simulink model "project3"  (R2022b)
settings: Solver=ode4  StartTime=0.0  StopTime=60  FixedStep=0.01  RelTol=1e-3
values from neighbouring files (symbols this model uses):
  Cd = 0.4    [project3_data.m]
  D_ref = 45    [project3_data.m]
  F_grade_const = M * g * sin(theta_rad)    [project3_data.m]
  F_roll_const = Cr * M * g * cos(theta_rad)    [project3_data.m]
  gamma_x = 0.001    [project3_data.m]
  K00 = (F_roll_const + F_grade_const) / K_torque    [project3_data.m]
  K_gap = 0.25    [project3_data.m]
  K_torque = eta_tf * N_tf2 / r_tire    (= 7.93333333333)    [project3_data.m]
  Kr0 = M_eq / (K_torque * tau_m)    (= 189.075630252)    [project3_data.m]
  Kx0 = -M_eq / (K_torque * tau_m)    (= -189.075630252)    [project3_data.m]
  M_eq = M + Mr2    (= 1200)    [project3_data.m]
  tau_m = 0.8    [project3_data.m]
  Te_max = 600    [project3_data.m]
  Te_min = -500    [project3_data.m]
  v_cmd_max = 90/3.6    (= 25)    [project3_data.m]
  v_cmd_min = 0    [project3_data.m]
  vE0 = 50/3.6    (= 13.8888888889)    [project3_data.m]
  xE0 = 0    [project3_data.m]
  xL0 = d0    (= 60)    [project3_data.m]
settings Model: Creator=Forough  LastModifiedBy=Forough

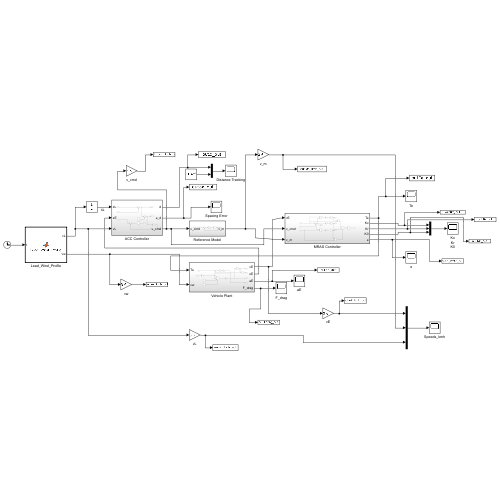
[thumbnail: Simulink's stored preview of the top-level diagram]
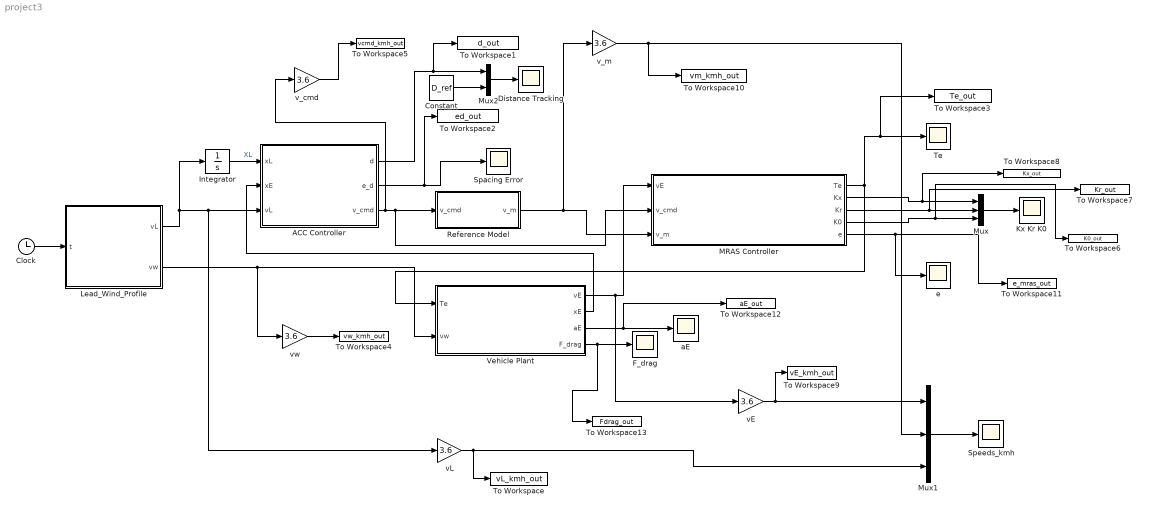
== system project3 ==
  ACC Controller : Subsystem
  Clock : Clock
  Constant : Constant  Value=D_ref
  Distance Tracking : Scope
  F_drag : Scope
  Integrator : Integrator  InitialCondition=xL0
  Kx Kr K0 : Scope
  Lead_Wind_Profile : MATLAB Function  TreatAsAtomicUnit=on
  MRAS Controller : Subsystem
  Mux : Mux  Inputs=3
  Mux1 : Mux  Inputs=3
  Mux2 : Mux  Inputs=2
  Reference Model : Subsystem
  Spacing Error : Scope
  "Speeds_kmh " : Scope
  Te : Scope
  To Workspace : ToWorkspace  VariableName=vL_kmh_out  SaveFormat=Timeseries  SampleTime=-1
  To Workspace1 : ToWorkspace  VariableName=d_out  SaveFormat=Timeseries  SampleTime=-1
  To Workspace10 : ToWorkspace  VariableName=vm_kmh_out  SaveFormat=Timeseries  SampleTime=-1
  To Workspace11 : ToWorkspace  VariableName=e_mras_out  SaveFormat=Timeseries  SampleTime=-1
  To Workspace12 : ToWorkspace  VariableName=aE_out  SaveFormat=Timeseries  SampleTime=-1
  To Workspace13 : ToWorkspace  VariableName=Fdrag_out  SaveFormat=Timeseries  SampleTime=-1
  To Workspace2 : ToWorkspace  VariableName=ed_out  SaveFormat=Timeseries  SampleTime=-1
  To Workspace3 : ToWorkspace  VariableName=Te_out  SaveFormat=Timeseries  SampleTime=-1
  To Workspace4 : ToWorkspace  VariableName=vw_kmh_out  SaveFormat=Timeseries  SampleTime=-1
  To Workspace5 : ToWorkspace  VariableName=vcmd_kmh_out  SaveFormat=Timeseries  SampleTime=-1
  To Workspace6 : ToWorkspace  VariableName=K0_out  SaveFormat=Timeseries  SampleTime=-1
  To Workspace7 : ToWorkspace  VariableName=Kr_out  SaveFormat=Timeseries  SampleTime=-1
  To Workspace8 : ToWorkspace  VariableName=Kx_out  SaveFormat=Timeseries  SampleTime=-1
  To Workspace9 : ToWorkspace  VariableName=vE_kmh_out  SaveFormat=Timeseries  SampleTime=-1
  Vehicle Plant : Subsystem
  aE : Scope
  e : Scope
  vE : Gain  Gain=3.6
  vL : Gain  Gain=3.6
  v_cmd : Gain  Gain=3.6
  v_m : Gain  Gain=3.6
  vw : Gain  Gain=3.6
  wires:
  Lead_Wind_Profile/1(vL) -> Integrator/1, vL/1, ACC Controller/3(vL)
  Integrator/1 -> ACC Controller/1(xL)  "XL"
  Lead_Wind_Profile/2(vw) -> vw/1, Vehicle Plant/2(vw)
  Clock/1 -> Lead_Wind_Profile/1(t)
  Vehicle Plant/2(xE) -> ACC Controller/2(xE)
  ACC Controller/3(v_cmd) -> v_cmd/1, MRAS Controller/2(v_cmd), Reference Model/1(v_cmd)
  Vehicle Plant/1(vE) -> vE/1, MRAS Controller/1(vE)
  Reference Model/1(v_m) -> v_m/1, MRAS Controller/3(v_m)
  MRAS Controller/1(Te) -> Vehicle Plant/1(Te), To Workspace3/1, Te/1
  MRAS Controller/2(Kx) -> To Workspace8/1, Mux/1
  MRAS Controller/3(Kr) -> To Workspace7/1, Mux/2
  MRAS Controller/4(K0) -> To Workspace6/1, Mux/3
  Mux/1 -> Kx Kr K0/1
  MRAS Controller/5(e) -> To Workspace11/1, e/1
  v_m/1 -> To Workspace10/1, Mux1/2
  vE/1 -> To Workspace9/1, Mux1/1
  vL/1 -> To Workspace/1, Mux1/3
  Mux1/1 -> "Speeds_kmh "/1
  ACC Controller/1(d) -> To Workspace1/1, Mux2/1
  Constant/1 -> Mux2/2
  Mux2/1 -> Distance Tracking/1
  ACC Controller/2(e_d) -> To Workspace2/1, Spacing Error/1
  Vehicle Plant/3(aE) -> To Workspace12/1, aE/1
  Vehicle Plant/4(F_drag) -> To Workspace13/1, F_drag/1
  vw/1 -> To Workspace4/1
  v_cmd/1 -> To Workspace5/1

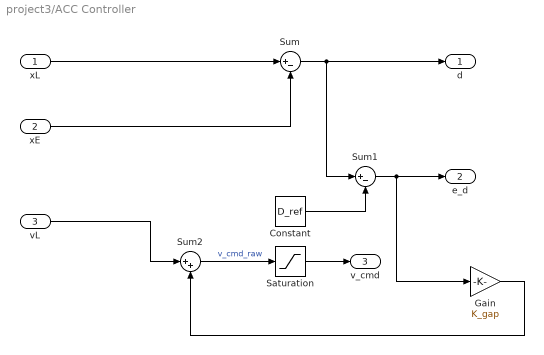
== system project3/ACC Controller ==
  xL : Inport
  xE : Inport  Port=2
  vL : Inport  Port=3
  Constant : Constant  Value=D_ref
  Gain : Gain  Gain=K_gap
  Saturation : Saturate  UpperLimit=v_cmd_max  LowerLimit=v_cmd_min
  Sum : Sum  Inputs=|+-
  Sum1 : Sum  Inputs=|+-
  Sum2 : Sum  Inputs=|++
  d : Outport
  e_d : Outport  Port=2
  v_cmd : Outport  Port=3
  wires:
  xL/1 -> Sum/1
  xE/1 -> Sum/2
  Sum/1 -> Sum1/1, d/1
  Constant/1 -> Sum1/2
  Sum1/1 -> Gain/1, e_d/1
  Gain/1 -> Sum2/2
  vL/1 -> Sum2/1
  Sum2/1 -> Saturation/1  "v_cmd_raw"
  Saturation/1 -> v_cmd/1

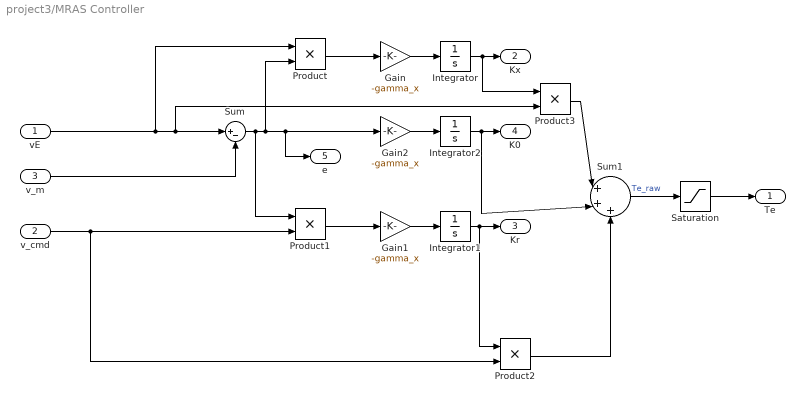
== system project3/MRAS Controller ==
  vE : Inport
  v_cmd : Inport  Port=2
  v_m : Inport  Port=3
  Gain : Gain  Gain=-gamma_x
  Gain1 : Gain  Gain=-gamma_x
  Gain2 : Gain  Gain=-gamma_x
  Integrator : Integrator  InitialCondition=Kx0
  Integrator1 : Integrator  InitialCondition=Kr0
  Integrator2 : Integrator  InitialCondition=K00
  Product{,1..3} (4 alike) : Product
  Saturation : Saturate  UpperLimit=Te_max  LowerLimit=Te_min  LinearizeAsGain=off
  Sum : Sum  Inputs=|+-
  Sum1 : Sum  Inputs=|+++
  Te : Outport
  Kx : Outport  Port=2
  Kr : Outport  Port=3
  K0 : Outport  Port=4
  e : Outport  Port=5
  wires:
  vE/1 -> Product/1, Product3/2, Sum/1
  v_m/1 -> Sum/2
  Sum/1 -> Product1/1, Product/2, Gain2/1, e/1
  Product/1 -> Gain/1
  Gain/1 -> Integrator/1
  Integrator/1 -> Product3/1, Kx/1
  Gain1/1 -> Integrator1/1
  Product1/1 -> Gain1/1
  Integrator1/1 -> Product2/1, Kr/1
  v_cmd/1 -> Product2/2, Product1/2
  Gain2/1 -> Integrator2/1
  Integrator2/1 -> Sum1/2, K0/1
  Product3/1 -> Sum1/1
  Product2/1 -> Sum1/3
  Sum1/1 -> Saturation/1  "Te_raw"
  Saturation/1 -> Te/1

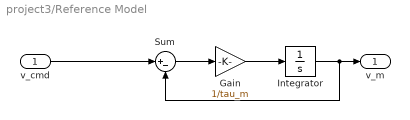
== system project3/Reference Model ==
  v_cmd : Inport
  Gain : Gain  Gain=1/tau_m
  Integrator : Integrator  InitialCondition=vE0
  Sum : Sum  Inputs=|+-
  v_m : Outport
  wires:
  v_cmd/1 -> Sum/1
  Sum/1 -> Gain/1
  Gain/1 -> Integrator/1
  Integrator/1 -> Sum/2, v_m/1

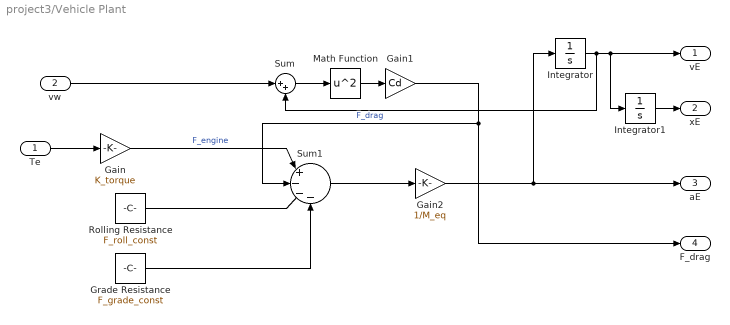
== system project3/Vehicle Plant ==
  Te : Inport
  vw : Inport  Port=2
  Gain : Gain  Gain=K_torque
  Gain1 : Gain  Gain=Cd
  Gain2 : Gain  Gain=1/M_eq
  Grade Resistance : Constant  Value=F_grade_const
  Integrator : Integrator  InitialCondition=vE0  LimitOutput=on  LowerSaturationLimit=0
  Integrator1 : Integrator  InitialCondition=xE0
  Math Function : Math  Operator=square
  Rolling Resistance : Constant  Value=F_roll_const
  Sum : Sum  Inputs=|++
  Sum1 : Sum  Inputs=|+---
  vE : Outport
  xE : Outport  Port=2
  aE : Outport  Port=3
  F_drag : Outport  Port=4
  wires:
  Te/1 -> Gain/1
  Gain/1 -> Sum1/1  "F_engine"
  vw/1 -> Sum/1
  Sum/1 -> Math Function/1
  Math Function/1 -> Gain1/1
  Gain1/1 -> Sum1/2, F_drag/1  "F_drag"
  Rolling Resistance/1 -> Sum1/3
  Grade Resistance/1 -> Sum1/4
  Sum1/1 -> Gain2/1
  Gain2/1 -> Integrator/1, aE/1
  Integrator/1 -> Sum/2, Integrator1/1, vE/1
  Integrator1/1 -> xE/1

== matlab function project3/Lead_Wind_Profile ==
  data: t input; vL output; vw output
function [vL, vw] = Lead_Wind_Profile(t)

% Lead vehicle speed profile:
% 10 km/h -> 15 km/h in first 15 s
% 15 km/h -> 20 km/h in next 15 s

if t <= 15
    vL_kmh = 10 + (15 - 10)/15 * t;
else
    vL_kmh = 15 + (20 - 15)/15 * (t - 15);
end

if vL_kmh > 20
    vL_kmh = 20;
end

% Head wind speed profile:
% 50 km/h -> 80 km/h in 30 s

vw_kmh = 50 + (80 - 50)/30 * t;

if vw_kmh > 80
    vw_kmh = 80;
end

% Convert km/h to m/s
vL = vL_kmh / 3.6;
vw = vw_kmh / 3.6;

end
